simulink model "BungeeJumping"  (R2020a)
settings: Solver=VariableStepAuto  StartTime=0.0  StopTime=100  RelTol=1e-6
undefined symbols (not defined in the file or in its folder): a1, a2, g, k, m
settings Model: Creator=faith  LastModifiedBy=faith

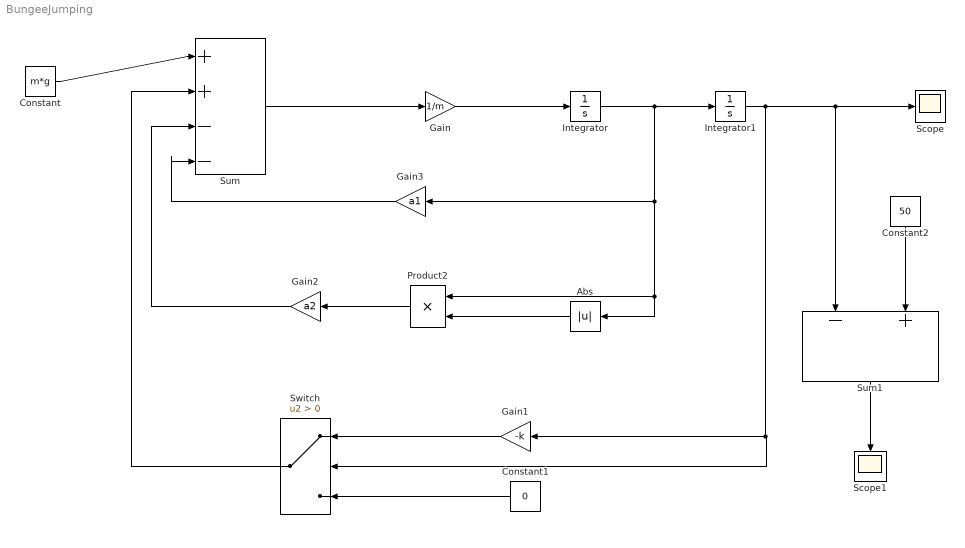
== system BungeeJumping ==
  Abs : Abs
  Constant : Constant  Value=m*g
  Constant1 : Constant  Value=0
  Constant2 : Constant  Value=50
  Gain : Gain  Gain=1/m
  Gain1 : Gain  Gain=-k
  Gain2 : Gain  Gain=a2
  Gain3 : Gain  Gain=a1
  Integrator : Integrator
  Integrator1 : Integrator  InitialCondition=-30
  Product2 : Product
  Scope : Scope
  Scope1 : Scope
  Sum : Sum  Inputs=|++--
  Sum1 : Sum  Inputs=-+
  Switch : Switch  Criteria=u2 > Threshold
  wires:
  Integrator/1 -> Gain3/1, Abs/1, Product2/1, Integrator1/1
  Gain/1 -> Integrator/1
  Sum/1 -> Gain/1
  Integrator1/1 -> Scope/1, Sum1/1, Gain1/1, Switch/2
  Switch/1 -> Sum/2
  Constant/1 -> Sum/1
  Gain1/1 -> Switch/1
  Constant1/1 -> Switch/3
  Abs/1 -> Product2/2
  Product2/1 -> Gain2/1
  Gain3/1 -> Sum/4
  Constant2/1 -> Sum1/2
  Sum1/1 -> Scope1/1
  Gain2/1 -> Sum/3
